simulink model "JoshTestingOCTModel"  (R2018b)
settings: Solver=VariableStepAuto  StartTime=0.0  StopTime=simParams.duration.Value  FixedStep=0.01  MaxStep=0.1*sqrt(simParams.lengthScaleFactor.Value)  RelTol=1e-3  AbsTol=1e-3
undefined symbols (not defined in the file): dragTurbine, dragTurbine_ul, env, flightController, FLIGHTCONTROLLER, flightController_cl, fltCtrl, fluidDynamicSurface, fluidDynamicSurface_cl, fuselage, fuselage_cl, initializeBussesFromBlock, initializeVariantsFromBlock, pathFollowingController, pathFollowingController_cl, plant, plant_cl, sixDoFDynamics, sixDoFDynamics_cl, sixDoFDynamicsCoupled, surfaceCoefficients, surfaceCoefficients_ul, tethersMoment, tethersMoment_cl, thrAttachPtKinematics, thrAttachPtKinematics_ul, vehicle, vehicle_cl, vehicleLE, vehicleLE_cl, vhcl
libraries: vrlib x18, dspstat3 x3, vectorNormalizer_ul x3, localApparentWind_ul x3, xProdMatrix_ul x2, dynamicPressure_ul x2, dsppolyfun x2, animation_cl x1, environment_cl x1, oneTetherThreeSurfaceCtrl_cl x1, courseFollow_cl x1, ctrlAllocMatrixLE_cl x1
(part 2 of 2)

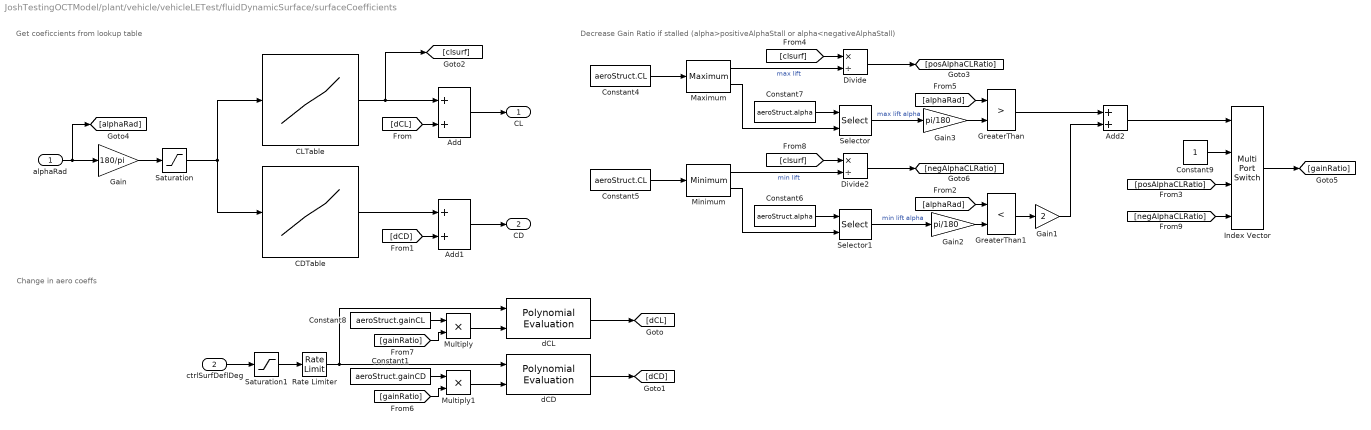
== system JoshTestingOCTModel/plant/vehicle/vehicleLETest/fluidDynamicSurface/surfaceCoefficients ==
  note: Get coeficcients from lookup table
  note: Decrease Gain Ratio if stalled (alpha>positiveAlphaStall or alpha<negativeAlphaStall)
  note: Change in aero coeffs
  alphaRad : Inport
  ctrlSurfDeflDeg : Inport  Port=2
  Add : Sum
  Add1 : Sum
  Add2 : Sum
  CDTable : Lookup_n-D  NumberOfTableDimensions=1  LookupTableObject=CLTable  BreakpointsForDimension1=aeroStruct.alpha  Table=aeroStruct.CD  ExtrapMethod=Clip  UseLastTableValue=on  InternalRulePriority=Speed  RndMeth=Simplest  InputSameDT=on
  CLTable : Lookup_n-D  NumberOfTableDimensions=1  LookupTableObject=CLTable  BreakpointsForDimension1=aeroStruct.alpha  Table=aeroStruct.CL  ExtrapMethod=Clip  UseLastTableValue=on  InternalRulePriority=Speed  RndMeth=Simplest  InputSameDT=on
  Constant1 : Constant  Value=aeroStruct.gainCD
  Constant4 : Constant  Value=aeroStruct.CL
  Constant5 : Constant  Value=aeroStruct.CL
  Constant6 : Constant  Value=aeroStruct.alpha
  Constant7 : Constant  Value=aeroStruct.alpha
  Constant8 : Constant  Value=aeroStruct.gainCL
  Constant9 : Constant
  Divide : Product  Inputs=*/
  Divide2 : Product  Inputs=*/
  Gain : Gain  Gain=180/pi
  Gain1 : Gain  Gain=2
  Gain2 : Gain  Gain=pi/180
  Gain3 : Gain  Gain=pi/180
  GreaterThan : RelationalOperator  Operator=>  OutDataTypeStr=boolean  RndMeth=Simplest
  GreaterThan1 : RelationalOperator  Operator=<  OutDataTypeStr=boolean  RndMeth=Simplest
  Index Vector : MultiPortSwitch  DataPortOrder=Zero-based contiguous  zeroidx=on
  Maximum : dspstat3/Maximum  operation=maximum  fcn=Value and Index  indexBase=One  operateOver=Each column  Dimension=1  InputProcessing=Columns as channels (frame based)  reset=None  roiEnable=off  roiType=Rectangles  roiPortion=Entire ROI  roiOutput=Individual statistics for each ROI  roiFlag=off  roundingMode=Floor  overflowMode=off  accumDataTypeStr=Inherit: Same as product output  accumLastDataTypeStr=Inherit: Same as product output
  Minimum : dspstat3/Minimum  operation=minimum  fcn=Value and Index  indexBase=One  operateOver=Each column  Dimension=1  InputProcessing=Columns as channels (frame based)  reset=None  roiEnable=off  roiType=Rectangles  roiPortion=Entire ROI  roiOutput=Individual statistics for each ROI  roiFlag=off  roundingMode=Floor  overflowMode=off
      settings: SourceProductName=DSP System Toolbox  SourceProductBaseCode=DS
  Multiply : Product
  Multiply1 : Product
  Rate Limiter : RateLimiter  RisingSlewLimit=aeroStruct.maxCtrlDefSpeed  FallingSlewLimit=-aeroStruct.maxCtrlDefSpeed  SampleTimeMode=inherited
  Saturation : Saturate  UpperLimit=90  LowerLimit=-90
  Saturation1 : Saturate  UpperLimit=aeroStruct.maxCtrlDef  LowerLimit=aeroStruct.minCtrlDef
  Selector : Selector  InputPortWidth=length(vhcl.portWing.alpha.Value)  IndexOptions=Index vector (port)  Indices=[1 3]  OutputSizes=1
  Selector1 : Selector  InputPortWidth=length(vhcl.portWing.alpha.Value)  IndexOptions=Index vector (port)  Indices=[1 3]  OutputSizes=1
  dCD : dsppolyfun/Polynomial Evaluation  useConstCoeffs=off  constCoeffs=[0]
      settings: SourceProductName=DSP System Toolbox  SourceProductBaseCode=DS
  dCL : dsppolyfun/Polynomial Evaluation  useConstCoeffs=off  constCoeffs=[0]
      settings: SourceProductName=DSP System Toolbox  SourceProductBaseCode=DS
  CL : Outport
  CD : Outport  Port=2
  wires:
  Gain/1 -> Saturation/1
  dCL/1 -> [dCL]
  dCD/1 -> [dCD]
  [dCL] -> Add/2
  CLTable/1 -> [clsurf], Add/1
  Add/1 -> CL/1
  Add1/1 -> CD/1
  [dCD] -> Add1/2
  CDTable/1 -> Add1/1
  Multiply1/1 -> dCD/2
  Rate Limiter/1 -> dCL/1, dCD/1
  ctrlSurfDeflDeg/1 -> Saturation1/1
  Saturation/1 -> CLTable/1, CDTable/1
  Constant4/1 -> Maximum/1
  alphaRad/1 -> [alphaRad], Gain/1
  Constant7/1 -> Selector/1
  Maximum/2 -> Selector/2
  Selector/1 -> Gain3/1  "max lift alpha"
  Divide/1 -> [posAlphaCLRatio]
  Maximum/1 -> Divide/2  "max lift"
  [clsurf] -> Divide/1
  [alphaRad] -> GreaterThan/1
  Minimum/2 -> Selector1/2
  [clsurf] -> Divide2/1
  Divide2/1 -> [negAlphaCLRatio]
  Minimum/1 -> Divide2/2  "min lift"
  Constant6/1 -> Selector1/1
  Constant5/1 -> Minimum/1
  Selector1/1 -> Gain2/1  "min lift alpha"
  [alphaRad] -> GreaterThan1/1
  GreaterThan1/1 -> Gain1/1
  GreaterThan/1 -> Add2/1
  Gain1/1 -> Add2/2
  Add2/1 -> Index Vector/1
  Constant9/1 -> Index Vector/2
  [negAlphaCLRatio] -> Index Vector/4
  [posAlphaCLRatio] -> Index Vector/3
  Index Vector/1 -> [gainRatio]
  Constant8/1 -> Multiply/1
  [gainRatio] -> Multiply/2
  Multiply/1 -> dCL/2
  [gainRatio] -> Multiply1/2
  Constant1/1 -> Multiply1/1
  Gain2/1 -> GreaterThan1/2
  Gain3/1 -> GreaterThan/2
  Saturation1/1 -> Rate Limiter/1

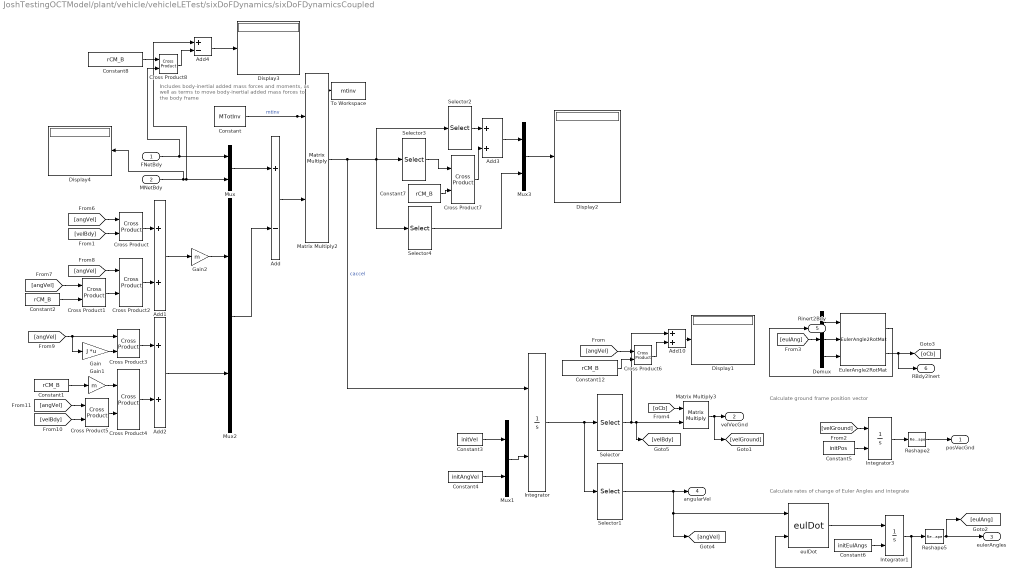
== system JoshTestingOCTModel/plant/vehicle/vehicleLETest/sixDoFDynamics/sixDoFDynamicsCoupled ==
  note: Includes body-inertial added mass forces and moments,
      | as well as terms to move body-inertial added mass
      | forces to the body frame
  note: Calculate ground frame position vector
  note: Calculate rates of change of Euler Angles and integrate
  FNetBdy : Inport
  MNetBdy : Inport  Port=2
  Add : Sum  Inputs=+-
  Add{1..3,10} (4 alike) : Sum
  Add4 : Sum  Inputs=+-
  Constant : Constant  Value=MTotInv  VectorParams1D=off
  Constant{1..2,7..8,12} (5 alike) : Constant  Value=rCM_B
  Constant3 : Constant  Value=initVel
  Constant4 : Constant  Value=initAngVel
  Constant5 : Constant  Value=initPos
  Constant6 : Constant  Value=initEulAngs
  Cross Product{,1..8} (9 alike) : vrlib/Utilities/Cross Product
      settings: SourceProductBaseCode=VR
  Demux : Demux  Outputs=3
  Display{1..4} (4 alike) : Display
  EulerAngle2RotMat : eulAng2RotMat_ul/EulerAngle2RotMat  SystemSampleTime=-1
  Gain : Gain  Gain=J  Multiplication=Matrix(K*u)
  Gain1 : Gain  Gain=m
  Gain2 : Gain  Gain=m
  Integrator : Integrator  InitialConditionSource=external
  Integrator1 : Integrator  InitialConditionSource=external  InitialCondition=initEulAngs
  Integrator3 : Integrator  InitialConditionSource=external  InitialCondition=initPos
  Matrix Multiply2 : Product  Multiplication=Matrix(*)
  Matrix Multiply3 : Product  Multiplication=Matrix(*)
  Mux{,1..3} (4 alike) : Mux  Inputs=2
  Reshape2 : Reshape  OutputDimensionality=Column vector (2-D)
  Reshape5 : Reshape  OutputDimensionality=Column vector (2-D)
  Selector : Selector  InputPortWidth=6  IndexOptions=Index vector (dialog)  Indices=[1 2 3]  OutputSizes=1
  Selector1 : Selector  InputPortWidth=6  IndexOptions=Index vector (dialog)  Indices=[4 5 6]  OutputSizes=1
  Selector2 : Selector  InputPortWidth=6  IndexOptions=Index vector (dialog)  Indices=[1 2 3]  OutputSizes=1
  Selector3 : Selector  InputPortWidth=6  IndexOptions=Index vector (dialog)  Indices=[4 5 6]  OutputSizes=1
  Selector4 : Selector  InputPortWidth=6  IndexOptions=Index vector (dialog)  Indices=[4 5 6]  OutputSizes=1
  To Workspace : ToWorkspace  VariableName=mtinv  SaveFormat=Timeseries  SampleTime=-1
  eulDot : eulDot/eulDot  SystemSampleTime=-1
  posVecGnd : Outport
  velVecGnd : Outport  Port=2
  eulerAngles : Outport  Port=3
  angularVel : Outport  Port=4
  Rinert2Bdy : Outport  Port=5
  RBdy2Inert : Outport  Port=6
  wires:
  Mux/1 -> Add/1
  Constant/1 -> To Workspace/1, Matrix Multiply2/1  "mtinv"
  Matrix Multiply2/1 -> Integrator/1, Selector4/1, Selector3/1, Selector2/1  "caccel"
  Integrator/1 -> Selector1/1, Selector/1
  Constant4/1 -> Mux1/2
  Mux1/1 -> Integrator/2
  Integrator3/1 -> Reshape2/1
  Demux/3 -> EulerAngle2RotMat/3
  Demux/1 -> EulerAngle2RotMat/1
  EulerAngle2RotMat/2 -> RBdy2Inert/1, [oCb]
  Reshape2/1 -> posVecGnd/1
  Demux/2 -> EulerAngle2RotMat/2
  Constant5/1 -> Integrator3/2
  [eulAng] -> Demux/1
  eulDot/1 -> Integrator1/1
  Integrator1/1 -> Reshape5/1, eulDot/2
  Constant6/1 -> Integrator1/2
  Reshape5/1 -> eulerAngles/1, [eulAng]
  Selector1/1 -> [angVel], eulDot/1, angularVel/1
  [velGround] -> Integrator3/1
  EulerAngle2RotMat/1 -> Rinert2Bdy/1
  Constant3/1 -> Mux1/1
  [oCb] -> Matrix Multiply3/1
  Matrix Multiply3/1 -> [velGround], velVecGnd/1
  Mux2/1 -> Add/2
  [velBdy] -> Cross Product/2
  [angVel] -> Cross Product/1
  Cross Product/1 -> Add1/1
  Cross Product1/1 -> Cross Product2/2
  Constant2/1 -> Cross Product1/2
  [angVel] -> Cross Product1/1
  [angVel] -> Cross Product2/1
  Cross Product2/1 -> Add1/2
  [angVel] -> Cross Product3/1, Gain/1
  Gain/1 -> Cross Product3/2
  Constant1/1 -> Gain1/1
  Gain1/1 -> Cross Product4/1
  [velBdy] -> Cross Product5/2
  [angVel] -> Cross Product5/1
  Cross Product5/1 -> Cross Product4/2
  Cross Product3/1 -> Add2/1
  Cross Product4/1 -> Add2/2
  Add1/1 -> Gain2/1
  Add2/1 -> Mux2/2
  FNetBdy/1 -> Cross Product8/2, Mux/1
  Add/1 -> Matrix Multiply2/2
  Gain2/1 -> Mux2/1
  Add10/1 -> Display1/1
  Cross Product6/1 -> Add10/2
  [angVel] -> Cross Product6/1
  Selector/1 -> Add10/1, [velBdy], Matrix Multiply3/2
  Constant12/1 -> Cross Product6/2
  Cross Product7/1 -> Add3/2
  Selector3/1 -> Cross Product7/1
  Constant7/1 -> Cross Product7/2
  Selector2/1 -> Add3/1
  Add4/1 -> Display3/1
  Cross Product8/1 -> Add4/2
  MNetBdy/1 -> Display4/1, Add4/1, Mux/2
  Constant8/1 -> Cross Product8/1
  Add3/1 -> Mux3/1
  Mux3/1 -> Display2/1
  Selector4/1 -> Mux3/2

== system JoshTestingOCTModel/plant/vehicle/vehicleLETest/tethersMoment/moment ==
  forceInrtFrm : Inport
  mmtArmBdyFrm : Inport  Port=2
  inrt2BdyFrm : Inport  Port=3
  Cross Product : vrlib/Utilities/Cross Product
      settings: SourceProductBaseCode=VR
  Multiply : Product  Multiplication=Matrix(*)
  Reshape : Reshape  OutputDimensionality=Column vector (2-D)
  Reshape1 : Reshape  OutputDimensionality=Column vector (2-D)
  mmtVecBdyFrm : Outport
  wires:
  forceInrtFrm/1 -> Reshape/1
  inrt2BdyFrm/1 -> Multiply/1
  Multiply/1 -> Cross Product/2
  mmtArmBdyFrm/1 -> Reshape1/1
  Cross Product/1 -> mmtVecBdyFrm/1
  Reshape/1 -> Multiply/2
  Reshape1/1 -> Cross Product/1
